simulink model "ueb1_A1_b_ver3"  (R2016a)
settings: Solver=VariableStepAuto  StartTime=0.0  StopTime=10.0  MaxStep=0.05  RelTol=1e-3
values from neighbouring files (symbols this model uses):
  A = [ ... (first row only)    [ueb1.m]
settings Model: Creator=bachman0  LastModifiedBy=bachman0

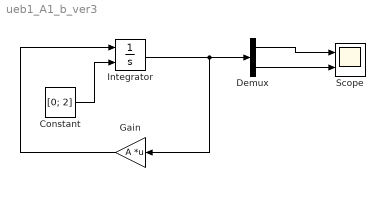
== system ueb1_A1_b_ver3 ==
  Constant : Constant  Value=[0; 2]
  Demux : Demux  Outputs=2
  Gain : Gain  Gain=A  Multiplication=Matrix(K*u)
  Integrator : Integrator  InitialConditionSource=external
  Scope : Scope  NumInputPorts=2
  wires:
  Gain/1 -> Integrator/1
  Constant/1 -> Integrator/2
  Integrator/1 -> Gain/1, Demux/1
  Demux/1 -> Scope/1
  Demux/2 -> Scope/2
